simulink model "exportFcnCode"  (R2024b)
settings: Solver=FixedStepAuto  StartTime=0.0  StopTime=10.0  RelTol=1e-3  EnableMultiTasking=on
PostLoadFcn:
  | Variant = 2;
undefined symbols (not defined in the file): CRANK_ANGLE_MAX_IGN, CRANK_ANGLES, cruiseRPM, cyl, duration, dwellAngle, enableCruiseControl, idleRPM, setIgnitionSchedule, timeout, writeCrankAngle, writeCrankRev, writeTotalRevs
libraries: simulink x3
CloseFcn:
  | clear Variant;
settings Model: PauseTimes=74.4  Creator=The MathWorks, Inc.  LastModifiedBy=grouleau
settings SolverCC: AlgebraicLoopSolver=TrustRegion
settings DataIOCC: ReturnWorkspaceOutputs=off
settings OptimizationCC: DefaultParameterBehavior=Inlined  PassReuseOutputArgsAs=Individual arguments  MaxStackSize=64  EfficientTunableParamExpr=on
settings DebuggingCC: ParameterTunabilityLossMsg=error  UnconnectedInputMsg=warning  UnconnectedOutputMsg=warning  UnconnectedLineMsg=warning  PregeneratedLibrarySubsystemCodeDiagnostic=none  ArithmeticOperatorsInVariantConditions=warning
settings HardwareCC: ProdBitPerPointer=32  ProdBitPerSizeT=32  ProdBitPerPtrDiffT=32  ProdLargestAtomicInteger=Long  ProdLargestAtomicFloat=Double  ProdWordSize=32  ProdHWDeviceType=ARM Compatible->ARM Cortex
settings ModelReferenceCC: EnableRefExpFcnMdlSchedulingChecks=on  ModelReferenceNumInstancesAllowed=Single
settings SFSimCC: SimUseLocalCustomCode=off  MATLABDynamicMemAlloc=off  CustomCodeUndefinedFunction=UseInterfaceOnly
settings RTWCC: Description=Embedded Coder  SystemTargetFile=ert.tlc  GenCodeOnly=on  TemplateMakefile=ert_default_tmf  GenerateReport=on  RTWUseLocalCustomCode=off  IncludeHyperlinkInReport=on  LaunchReport=on  GenerateTraceInfo=on  GenerateTraceReport=on  GenerateTraceReportSl=on  GenerateTraceReportSf=on  GenerateTraceReportEml=on  GPUComputeCapability=3.5
settings CodeAppCC: ForceParamTrailComments=on  IgnoreCustomStorageClasses=off  MaxIdLength=63  OperatorAnnotations=on  SimulinkDataObjDesc=on  SFDataObjDesc=on  InsertBlockDesc=on
settings ERTTargetCC: SupportVariableSizeSignals=on  InlinedParameterPlacement=Hierarchical  ERTCustomFileTemplate=example_file_process.tlc  DynamicArrayContainerType=coder::array

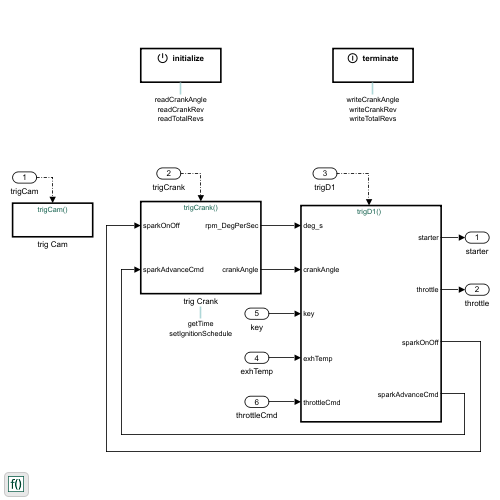
[thumbnail: Simulink's stored preview of the top-level diagram]
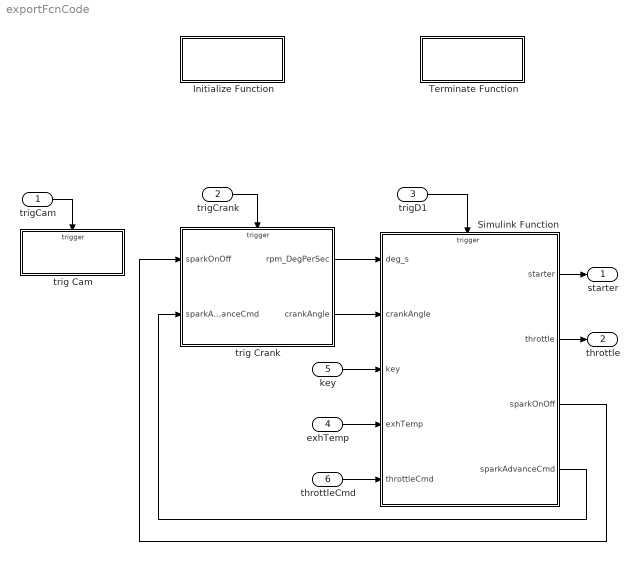
== system exportFcnCode ==
  trigCam : Inport  OutputFunctionCall=on
  trigCrank : Inport  Port=2  OutputFunctionCall=on
  trigD1 : Inport  Port=3  SampleTime=0.008  OutputFunctionCall=on
  exhTemp : Inport  Port=4
  key : Inport  Port=5
  throttleCmd : Inport  Port=6
  Initialize Function : Subsystem  TreatAsAtomicUnit=on
  Simulink Function : Subsystem  TreatAsAtomicUnit=on
  Terminate Function : Subsystem  TreatAsAtomicUnit=on
  trig Cam : Subsystem  TreatAsAtomicUnit=on
  trig Crank : Subsystem  TreatAsAtomicUnit=on
  starter : Outport  VectorParamsAs1DForOutWhenUnconnected=off
  throttle : Outport  Port=2  VectorParamsAs1DForOutWhenUnconnected=off
  wires:
  trig Crank/2(crankAngle) -> Simulink Function/2(crankAngle)
  Simulink Function/2(throttle) -> throttle/1
  Simulink Function/1(starter) -> starter/1
  trigCam/1 -> trig Cam/Trigger
  trig Crank/1(rpm_DegPerSec) -> Simulink Function/1(deg_s)
  key/1 -> Simulink Function/3(key)
  trigCrank/1 -> trig Crank/Trigger
  exhTemp/1 -> Simulink Function/4(exhTemp)
  Simulink Function/3(sparkOnOff) -> trig Crank/1(sparkOnOff)
  Simulink Function/4(sparkAdvanceCmd) -> trig Crank/2(sparkAdvanceCmd)
  trigD1/1 -> Simulink Function/Trigger
  throttleCmd/1 -> Simulink Function/5(throttleCmd)

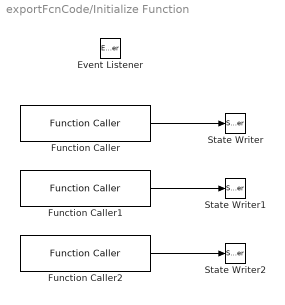
== system exportFcnCode/Initialize Function ==
  Event Listener : EventListener  DisableCoverage=on  EventName=reset
  Function Caller : FunctionCaller  FunctionPrototype=y = readCrankRev()  InputArgumentSpecifications=<Enter example>  OutputArgumentSpecifications=false
  Function Caller1 : FunctionCaller  FunctionPrototype=y = readTotalRevs()  InputArgumentSpecifications=<Enter example>  OutputArgumentSpecifications=0
  Function Caller2 : FunctionCaller  FunctionPrototype=y = readCrankAngle()  InputArgumentSpecifications=<Enter example>  OutputArgumentSpecifications=0
  State Writer : StateWriter  StateOwnerBlock=../../trig Crank/ManageRevolutions/crankRev  StateName=crankRev
  State Writer1 : StateWriter  StateOwnerBlock=../../trig Crank/ManageRevolutions/Total Crank Revolutions  StateName=totalCrankRevs
  State Writer2 : StateWriter  StateOwnerBlock=../../trig Crank/Count Teeth/Local Crank Angle
  wires:
  Function Caller/1 -> State Writer/1
  Function Caller2/1 -> State Writer2/1
  Function Caller1/1 -> State Writer1/1

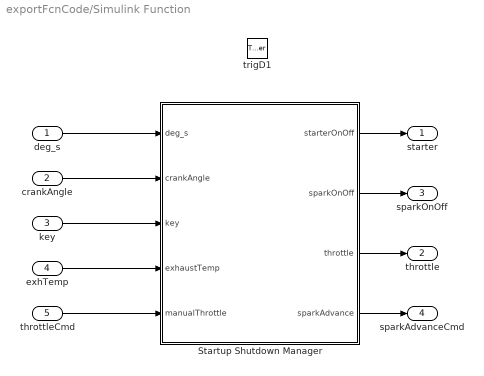
== system exportFcnCode/Simulink Function ==
  deg_s : Inport
  crankAngle : Inport  Port=2
  key : Inport  Port=3
  exhTemp : Inport  Port=4
  throttleCmd : Inport  Port=5
  trigD1 : TriggerPort  TriggerType=function-call  FunctionName=scheduleIgnition  FunctionVisibility=scoped  VariantControl=(inherit)  SampleTimeType=periodic  SampleTime=0.008
  Startup Shutdown Manager : Stateflow chart  TreatAsAtomicUnit=on
  starter : Outport  VectorParamsAs1DForOutWhenUnconnected=off
  throttle : Outport  Port=2  VectorParamsAs1DForOutWhenUnconnected=off
  sparkOnOff : Outport  Port=3  VectorParamsAs1DForOutWhenUnconnected=off
  sparkAdvanceCmd : Outport  Port=4  VectorParamsAs1DForOutWhenUnconnected=off
  wires:
  crankAngle/1 -> Startup Shutdown Manager/2(crankAngle)
  deg_s/1 -> Startup Shutdown Manager/1(deg_s)
  key/1 -> Startup Shutdown Manager/3(key)
  Startup Shutdown Manager/1(starterOnOff) -> starter/1
  Startup Shutdown Manager/2(sparkOnOff) -> sparkOnOff/1
  Startup Shutdown Manager/3(throttle) -> throttle/1
  exhTemp/1 -> Startup Shutdown Manager/4(exhaustTemp)
  Startup Shutdown Manager/4(sparkAdvance) -> sparkAdvanceCmd/1
  throttleCmd/1 -> Startup Shutdown Manager/5(manualThrottle)

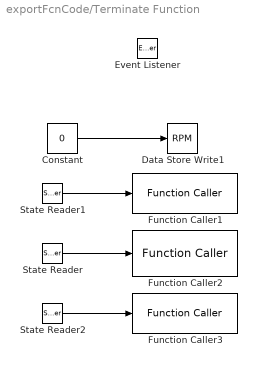
== system exportFcnCode/Terminate Function ==
  Constant : Constant  Value=0
  Data Store Write1 : DataStoreWrite  DataStoreName=RPM  IndexOptions=Index vector (dialog)  Indices=1  OutputSizes=1
  Event Listener : EventListener  DisableCoverage=on  EventType=Terminate  EventName=reset
  Function Caller1 : FunctionCaller  FunctionPrototype=writeCrankRev(u)  InputArgumentSpecifications=false  OutputArgumentSpecifications=<Enter example>
  Function Caller2 : FunctionCaller  FunctionPrototype=writeTotalRevs(u)  InputArgumentSpecifications=0  OutputArgumentSpecifications=<Enter example>
  Function Caller3 : FunctionCaller  FunctionPrototype=writeCrankAngle(u)  InputArgumentSpecifications=0  OutputArgumentSpecifications=<Enter example>
  State Reader : StateReader  StateOwnerBlock=../../trig Crank/ManageRevolutions/Total Crank Revolutions  StateName=totalCrankRevs
  State Reader1 : StateReader  StateOwnerBlock=../../trig Crank/ManageRevolutions/crankRev  StateName=crankRev
  State Reader2 : StateReader  StateOwnerBlock=../../trig Crank/Count Teeth/Local Crank Angle
  wires:
  State Reader/1 -> Function Caller2/1
  Constant/1 -> Data Store Write1/1
  State Reader2/1 -> Function Caller3/1
  State Reader1/1 -> Function Caller1/1

== system exportFcnCode/trig Cam ==
  trigCam : TriggerPort  TriggerType=function-call  FunctionName=trigCam  FunctionVisibility=scoped  VariantControl=(inherit)
  Constant : Constant  Value=false
  State Writer : StateWriter  StateOwnerBlock=../../trig Crank/ManageRevolutions/crankRev  StateName=crankRev
  wires:
  Constant/1 -> State Writer/1

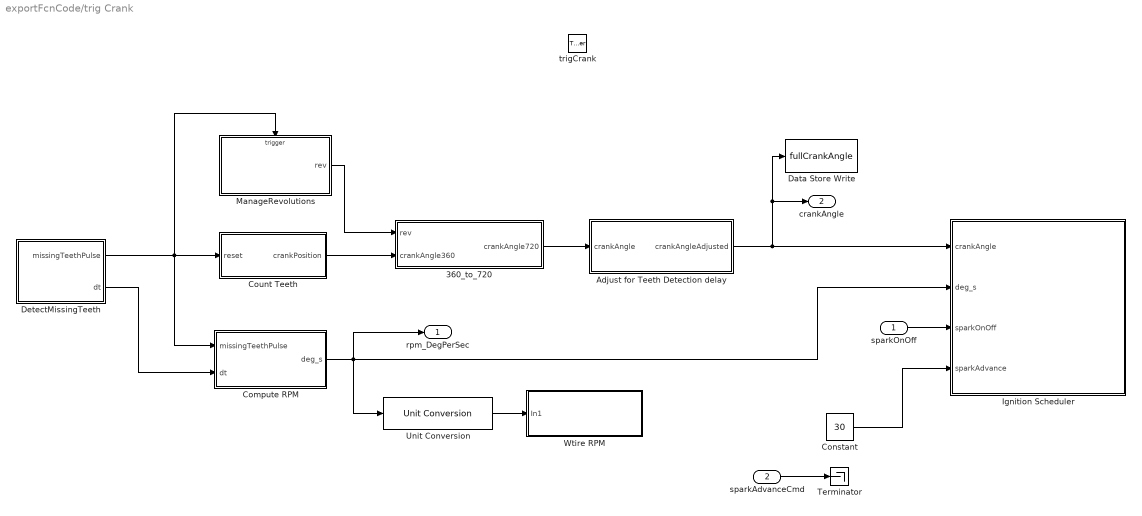
== system exportFcnCode/trig Crank ==
  sparkOnOff : Inport
  sparkAdvanceCmd : Inport  Port=2
  trigCrank : TriggerPort  TriggerType=function-call  FunctionName=trigCrank  FunctionVisibility=scoped  VariantControl=(inherit)
  360_to_720 : Subsystem
  Adjust for Teeth Detection delay : Subsystem
  Compute RPM : Subsystem
  Constant : Constant  Value=30
  Count Teeth : Subsystem
  Data Store Write : DataStoreWrite  DataStoreName=fullCrankAngle  IndexOptions=Index vector (dialog)  Indices=1  OutputSizes=1
  DetectMissingTeeth : Subsystem
  Ignition Scheduler : Stateflow chart  TreatAsAtomicUnit=on
  ManageRevolutions : Subsystem
  Terminator : Terminator
  Unit Conversion : UnitConversion
  Wtire RPM : Subsystem
  rpm_DegPerSec : Outport  VectorParamsAs1DForOutWhenUnconnected=off
  crankAngle : Outport  Port=2  VectorParamsAs1DForOutWhenUnconnected=off
  wires:
  360_to_720/1(crankAngle720) -> Adjust for Teeth Detection delay/1(crankAngle)
  Count Teeth/1(crankPosition) -> 360_to_720/2(crankAngle360)
  DetectMissingTeeth/1(missingTeethPulse) -> ManageRevolutions/Trigger, Compute RPM/1(missingTeethPulse), Count Teeth/1(reset)
  DetectMissingTeeth/2(dt) -> Compute RPM/2(dt)
  Compute RPM/1(deg_s) -> Ignition Scheduler/2(deg_s), Unit Conversion/1, rpm_DegPerSec/1
  Adjust for Teeth Detection delay/1(crankAngleAdjusted) -> Data Store Write/1, crankAngle/1, Ignition Scheduler/1(crankAngle)
  Unit Conversion/1 -> Wtire RPM/1(In1)
  sparkOnOff/1 -> Ignition Scheduler/3(sparkOnOff)
  ManageRevolutions/1(rev) -> 360_to_720/1(rev)
  Constant/1 -> Ignition Scheduler/4(sparkAdvance)
  sparkAdvanceCmd/1 -> Terminator/1

== system exportFcnCode/Simulink Function/Startup Shutdown Manager/ManageStartupShutdown.exhausttempCtrl ==
  exhTemp : Inport  OutDataTypeStr=double  PortDimensions=1
  f : TriggerPort  TriggerType=function-call  VariantControl=(inherit)
      settings: CopyFcn=Stateflow.SLINSF.SimulinkMan.removeBlockPreDeleteFcn  PreDeleteFcn=Stateflow.SLINSF.SimulinkMan.unsafePredeleteFcn
  1-D Lookup Table : Lookup_n-D  NumberOfTableDimensions=1  BreakpointsForDimension1=[25 50 75 100 150]  Table=[10 10 10 20 20]  ExtrapMethod=Clip  InternalRulePriority=Speed  RndMeth=Simplest
  sparkAdvance : Outport  VectorParamsAs1DForOutWhenUnconnected=off
  wires:
  exhTemp/1 -> 1-D Lookup Table/1
  1-D Lookup Table/1 -> sparkAdvance/1

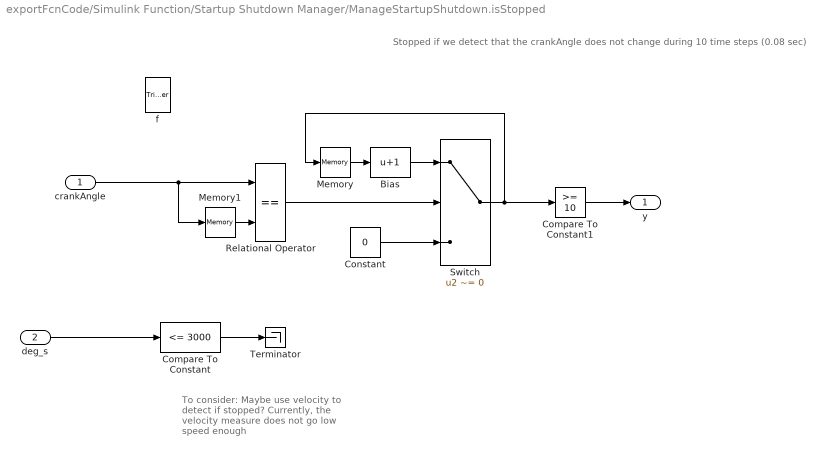
== system exportFcnCode/Simulink Function/Startup Shutdown Manager/ManageStartupShutdown.isStopped ==
  note: Stopped if we detect that the crankAngle does not change during 10 time steps (0.08 sec)
  note: To consider:
      | Maybe use velocity to detect if stopped?
      | Currently, the velocity measure does not go low speed enough
  crankAngle : Inport  OutDataTypeStr=double  PortDimensions=1
  deg_s : Inport  Port=2  OutDataTypeStr=double  PortDimensions=1
  f : TriggerPort  TriggerType=function-call  VariantControl=(inherit)
      settings: CopyFcn=Stateflow.SLINSF.SimulinkMan.removeBlockPreDeleteFcn  PreDeleteFcn=Stateflow.SLINSF.SimulinkMan.unsafePredeleteFcn
  Bias : Bias  Bias=1  SaturateOnIntegerOverflow=off
  Compare To Constant : simulink/Logic and Bit Operations/Compare To Constant  relop=<=  const=3000  OutDataTypeStr=boolean
  Compare To Constant1 : simulink/Logic and Bit Operations/Compare To Constant  relop=>=  const=10  OutDataTypeStr=boolean
  Constant : Constant  Value=0
  Memory : Memory  InheritSampleTime=on
  Memory1 : Memory  InheritSampleTime=on
  Relational Operator : RelationalOperator  Operator===  OutDataTypeStr=boolean  RndMeth=Simplest  InputSameDT=off
  Switch : Switch  Criteria=u2 ~= 0  SaturateOnIntegerOverflow=off  InputSameDT=off
  Terminator : Terminator
  y : Outport  OutDataTypeStr=boolean  PortDimensions=1  VectorParamsAs1DForOutWhenUnconnected=off
  wires:
  deg_s/1 -> Compare To Constant/1
  Switch/1 -> Compare To Constant1/1, Memory/1
  Memory/1 -> Bias/1
  Relational Operator/1 -> Switch/2
  crankAngle/1 -> Memory1/1, Relational Operator/1
  Bias/1 -> Switch/1
  Constant/1 -> Switch/3
  Memory1/1 -> Relational Operator/2
  Compare To Constant1/1 -> y/1
  Compare To Constant/1 -> Terminator/1

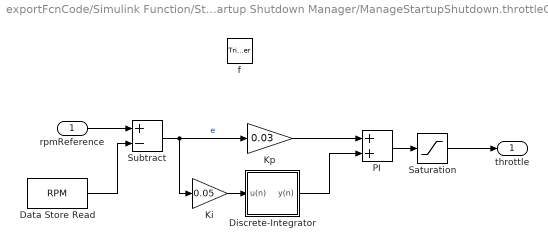
== system exportFcnCode/Simulink Function/Startup Shutdown Manager/ManageStartupShutdown.throttleControl ==
  rpmReference : Inport  OutDataTypeStr=double  PortDimensions=1
  f : TriggerPort  TriggerType=function-call  VariantControl=(inherit)
      settings: CopyFcn=Stateflow.SLINSF.SimulinkMan.removeBlockPreDeleteFcn  PreDeleteFcn=Stateflow.SLINSF.SimulinkMan.unsafePredeleteFcn
  Data Store Read : DataStoreRead  DataStoreName=RPM  IndexOptions=Index vector (dialog)  Indices=1  OutputSizes=1
  Discrete-Integrator : Subsystem
  Ki : Gain  Gain=0.05
  Kp : Gain  Gain=0.03
  PI : Sum
  Saturation : Saturate  UpperLimit=90  LowerLimit=0
  Subtract : Sum  Inputs=+-
  throttle : Outport  VectorParamsAs1DForOutWhenUnconnected=off
  wires:
  rpmReference/1 -> Subtract/1
  Data Store Read/1 -> Subtract/2
  Subtract/1 -> Kp/1, Ki/1  "e"
  Discrete-Integrator/1(y(n)) -> PI/2
  PI/1 -> Saturation/1
  Ki/1 -> Discrete-Integrator/1(u(n))
  Kp/1 -> PI/1
  Saturation/1 -> throttle/1

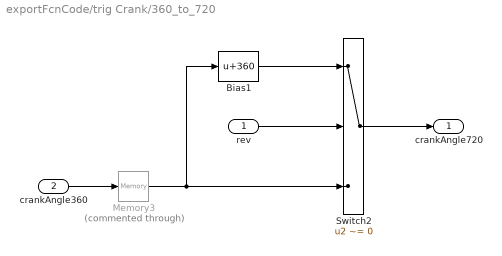
== system exportFcnCode/trig Crank/360_to_720 ==
  rev : Inport
  crankAngle360 : Inport  Port=2
  Bias1 : Bias  Bias=360  SaturateOnIntegerOverflow=off
  Memory3 : Memory  Commented=through  InheritSampleTime=on
  Switch2 : Switch  Criteria=u2 ~= 0  Threshold=34  SaturateOnIntegerOverflow=off  InputSameDT=off
  crankAngle720 : Outport  VectorParamsAs1DForOutWhenUnconnected=off
  wires:
  rev/1 -> Switch2/2
  Switch2/1 -> crankAngle720/1
  Bias1/1 -> Switch2/1
  Memory3/1 -> Bias1/1, Switch2/3
  crankAngle360/1 -> Memory3/1

== system exportFcnCode/trig Crank/Adjust for Teeth Detection delay ==
  crankAngle : Inport
  Bias2 : Bias  Commented=through  Bias=10  SaturateOnIntegerOverflow=off
  Bias3 : Bias  Bias=-710  SaturateOnIntegerOverflow=off
  Compare To Constant1 : simulink/Logic and Bit Operations/Compare To Constant  relop=>  const=700  OutDataTypeStr=boolean
  Switch3 : Switch  Criteria=u2 ~= 0  Threshold=34  SaturateOnIntegerOverflow=off  InputSameDT=off
  crankAngleAdjusted : Outport  VectorParamsAs1DForOutWhenUnconnected=off
  wires:
  Switch3/1 -> crankAngleAdjusted/1  "crankAngleAdjusted"
  Compare To Constant1/1 -> Switch3/2
  Bias2/1 -> Switch3/3, Compare To Constant1/1, Bias3/1
  crankAngle/1 -> Bias2/1
  Bias3/1 -> Switch3/1

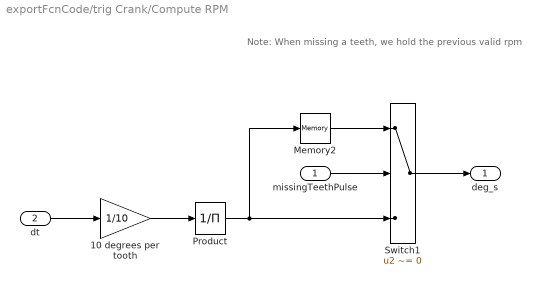
== system exportFcnCode/trig Crank/Compute RPM ==
  note: Note: When missing a teeth, we hold the previous valid rpm
  missingTeethPulse : Inport
  dt : Inport  Port=2  Unit=sec
  10 degrees per tooth : Gain  Gain=1/10
  Memory2 : Memory  InheritSampleTime=on
  Product : Product  Inputs=/
  Switch1 : Switch  Criteria=u2 ~= 0  Threshold=34  SaturateOnIntegerOverflow=off  InputSameDT=off
  deg_s : Outport  Unit=deg/sec  VectorParamsAs1DForOutWhenUnconnected=off
  wires:
  10 degrees per tooth/1 -> Product/1
  Product/1 -> Memory2/1, Switch1/3
  Memory2/1 -> Switch1/1
  Switch1/1 -> deg_s/1
  dt/1 -> 10 degrees per tooth/1
  missingTeethPulse/1 -> Switch1/2

== system exportFcnCode/trig Crank/Count Teeth ==
  note: Crank Position 0-360
  reset : Inport
  Bias : Bias  Bias=10  SaturateOnIntegerOverflow=off
  Constant1 : Constant  Value=0
  Local Crank Angle : UnitDelay  SampleTime=-1  HasFrameUpgradeWarning=on
  Switch : Switch  Criteria=u2 ~= 0  Threshold=34  SaturateOnIntegerOverflow=off  InputSameDT=off
  crankPosition : Outport  Unit=deg  VectorParamsAs1DForOutWhenUnconnected=off
  wires:
  Constant1/1 -> Switch/1
  reset/1 -> Switch/2
  Switch/1 -> Local Crank Angle/1, crankPosition/1
  Local Crank Angle/1 -> Bias/1
  Bias/1 -> Switch/3

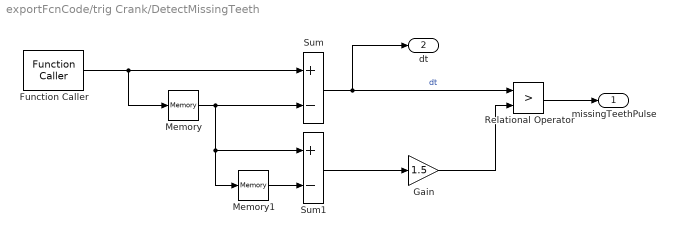
== system exportFcnCode/trig Crank/DetectMissingTeeth ==
  Function Caller : FunctionCaller  FunctionPrototype=y = getTime()  InputArgumentSpecifications=<Enter example>  OutputArgumentSpecifications=1
  Gain : Gain  Gain=1.5
  Memory : Memory  InheritSampleTime=on
  Memory1 : Memory  InheritSampleTime=on
  Relational Operator : RelationalOperator  Operator=>  OutDataTypeStr=boolean  RndMeth=Simplest  InputSameDT=off
  Sum : Sum  Inputs=+-
  Sum1 : Sum  Inputs=+-
  missingTeethPulse : Outport  VectorParamsAs1DForOutWhenUnconnected=off
  dt : Outport  Port=2  Unit=sec  VectorParamsAs1DForOutWhenUnconnected=off
  wires:
  Sum/1 -> dt/1, Relational Operator/1  "dt"
  Function Caller/1 -> Memory/1, Sum/1
  Memory/1 -> Sum1/1, Memory1/1, Sum/2
  Memory1/1 -> Sum1/2
  Relational Operator/1 -> missingTeethPulse/1
  Gain/1 -> Relational Operator/2
  Sum1/1 -> Gain/1

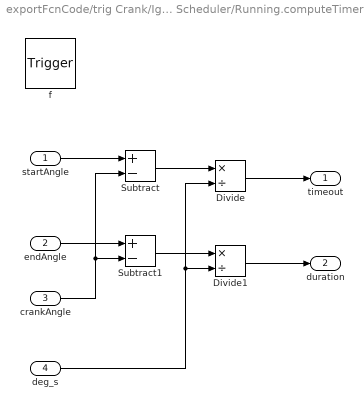
== system exportFcnCode/trig Crank/Ignition Scheduler/Running.computeTimerProps ==
  startAngle : Inport  OutDataTypeStr=double  PortDimensions=1
  endAngle : Inport  Port=2  OutDataTypeStr=double  PortDimensions=1
  crankAngle : Inport  Port=3  OutDataTypeStr=double  PortDimensions=1
  deg_s : Inport  Port=4  OutDataTypeStr=double  PortDimensions=1
  f : TriggerPort  TriggerType=function-call  VariantControl=(inherit)
      settings: CopyFcn=Stateflow.SLINSF.SimulinkMan.removeBlockPreDeleteFcn  PreDeleteFcn=Stateflow.SLINSF.SimulinkMan.unsafePredeleteFcn
  Divide : Product  Inputs=*/
  Divide1 : Product  Inputs=*/
  Subtract : Sum  Inputs=+-
  Subtract1 : Sum  Inputs=+-
  timeout : Outport  VectorParamsAs1DForOutWhenUnconnected=off
  duration : Outport  Port=2  VectorParamsAs1DForOutWhenUnconnected=off
  wires:
  startAngle/1 -> Subtract/1
  crankAngle/1 -> Subtract1/2, Subtract/2
  endAngle/1 -> Subtract1/1
  Subtract/1 -> Divide/1
  deg_s/1 -> Divide1/2, Divide/2
  Subtract1/1 -> Divide1/1
  Divide1/1 -> duration/1
  Divide/1 -> timeout/1

== system exportFcnCode/trig Crank/Ignition Scheduler/Running.setIgnitionScheduleWrapper ==
  cyl : Inport  OutDataTypeStr=double  PortDimensions=1
  timeout : Inport  Port=2  OutDataTypeStr=double  PortDimensions=1
  duration : Inport  Port=3  OutDataTypeStr=double  PortDimensions=1
  f : TriggerPort  TriggerType=function-call  VariantControl=(inherit)
      settings: CopyFcn=Stateflow.SLINSF.SimulinkMan.removeBlockPreDeleteFcn  PreDeleteFcn=Stateflow.SLINSF.SimulinkMan.unsafePredeleteFcn
  Function Caller : FunctionCaller  FunctionPrototype=setIgnitionSchedule(cyl,timeout,duration)  InputArgumentSpecifications=1,1,1  OutputArgumentSpecifications=<Enter example>
  wires:
  cyl/1 -> Function Caller/1
  timeout/1 -> Function Caller/2
  duration/1 -> Function Caller/3

== system exportFcnCode/trig Crank/ManageRevolutions ==
  Trigger : TriggerPort  VariantControl=Variant  PortDimensions=1
  Bias : Bias  Bias=1  SaturateOnIntegerOverflow=off
  NOT : Logic  Operator=NOT  IconShape=distinctive  AllPortsSameDT=off  OutDataTypeStr=boolean
  Total Crank Revolutions : UnitDelay  SampleTime=-1  StateName=totalCrankRevs  HasFrameUpgradeWarning=on
  crankRev : UnitDelay  InitialCondition=false  SampleTime=-1  StateName=crankRev  HasFrameUpgradeWarning=on
  rev : Outport  VectorParamsAs1DForOutWhenUnconnected=off
  wires:
  crankRev/1 -> NOT/1
  NOT/1 -> rev/1, crankRev/1
  Bias/1 -> Total Crank Revolutions/1
  Total Crank Revolutions/1 -> Bias/1

== system exportFcnCode/trig Crank/Wtire RPM ==
  In1 : Inport  Unit=rpm
  Data Store Write1 : DataStoreWrite  DataStoreName=RPM  IndexOptions=Index vector (dialog)  Indices=1  OutputSizes=1
  wires:
  In1/1 -> Data Store Write1/1

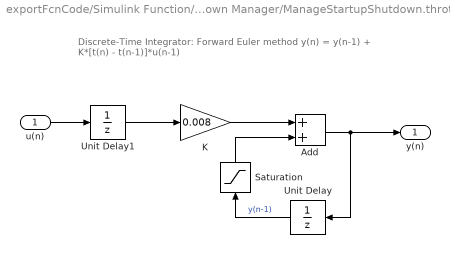
== system exportFcnCode/Simulink Function/Startup Shutdown Manager/ManageStartupShutdown.throttleControl/Discrete-Integrator ==
  note: Discrete-Time Integrator: Forward Euler method
      | y(n) = y(n-1) + K*[t(n) - t(n-1)]*u(n-1)
  u(n) : Inport
  Add : Sum
  K : Gain  Gain=0.008
  Saturation : Saturate  UpperLimit=90  LowerLimit=0
  Unit Delay : UnitDelay  SampleTime=-1  HasFrameUpgradeWarning=on
  Unit Delay1 : UnitDelay  SampleTime=-1  HasFrameUpgradeWarning=on
  y(n) : Outport  VectorParamsAs1DForOutWhenUnconnected=off
  wires:
  K/1 -> Add/1
  Unit Delay1/1 -> K/1
  Add/1 -> y(n)/1, Unit Delay/1
  u(n)/1 -> Unit Delay1/1
  Unit Delay/1 -> Saturation/1  "y(n-1)"
  Saturation/1 -> Add/2

== stateflow chart exportFcnCode/Simulink Function/Startup Shutdown Manager ==
  settings: sampleTime=0.008
  state ManageStartupShutdown [parallel]
    settings: executionOrder=1
    state Off
      entry: starterOnOff = false;
      sparkOnOff = false;
      throttle = 0;
    state Running
      state StarterOn
        entry: starterOnOff = true;
      state SparkOn
        entry: sparkOnOff = true;
        throttle = 90;
      state StarterAndEngine
      state StarterOff
        entry:
        starterOnOff = false;
        entry, during:
        if(enableCruiseControl)
        throttle = throttleControl(cruiseRPM);
        else
        throttle = manualThrottle+throttleControl(idleRPM);
        end
        sparkAdvance = exhausttempCtrl(exhaustTemp);
      (default) -> StarterOn
      StarterOn -> SparkOn : after(0.5,sec)
      SparkOn -> StarterAndEngine
      StarterAndEngine -> StarterOff : [deg_s>10000] % over 1600 RPM
    state WaitingForZeroSped
    state throttle = throttleControl(rpmReference) [function]
    state y = isStopped(crankAngle,deg_s) [function]
    state sparkAdvance = exhausttempCtrl(exhTemp) [function]
    (default) -> Off
    (junction 242) -> Off
    (junction 241) -> (junction 242) : [isStopped(crankAngle,deg_s)]
        | {isECUPowered = false;}
    Off -> Running : [key == true]
    Running -> WaitingForZeroSped : [key == false]
        | {throttle = 0;sparkOnOff=false}
    WaitingForZeroSped -> (junction 241)
  data: throttle function_output; rpmReference function_input double size=1; crankAngle function_input double size=1; deg_s function_input double size=1; y function_output boolean size=1; exhTemp function_input double size=1; sparkAdvance function_output; deg_s input; dwellAngle parameter; crankAngle input; CRANK_ANGLES parameter; key input boolean size=1; starterOnOff output boolean size=1; sparkOnOff output boolean size=1; throttle output double size=1; isECUPowered data_store_memory; enableCruiseControl parameter; cruiseRPM parameter; exhaustTemp input; idleRPM parameter; sparkAdvance output; manualThrottle input

== stateflow chart exportFcnCode/trig Crank/Ignition Scheduler ==
  state Wait
  state Running
    state [timeout, duration] = computeTimerProps(startAngle, endAngle, crankAngle, deg_s) [function]
    state setIgnitionScheduleWrapper(cyl,timeout,duration) [function]
    state WaitNextQuadrant
    note: CRANK_ANGLES = [720 180 360 540];
    state startAt1
      en:  endAngle = CRANK_ANGLES(1) - sparkAdvance;
      startAngle = endAngle-dwellAngle;
    state IgnitionCyl1
      entry: [timeout, duration] = computeTimerProps(startAngle, endAngle, crankAngle, deg_s);
      setIgnitionScheduleWrapper(1,timeout,duration);
      endAngle = CRANK_ANGLES(2) - sparkAdvance;
      startAngle = endAngle-dwellAngle;
    state IgnitionCyl2
      entry: [timeout, duration] = computeTimerProps(startAngle, endAngle, crankAngle, deg_s);
      setIgnitionScheduleWrapper(2,timeout,duration);
      endAngle = CRANK_ANGLES(3) - sparkAdvance;
      startAngle = endAngle-dwellAngle;
    state startAt2
      en:  endAngle = CRANK_ANGLES(2) - sparkAdvance;
      startAngle = endAngle-dwellAngle;
    state IgnitionCyl3
      entry: [timeout, duration] = computeTimerProps(startAngle, endAngle, crankAngle, deg_s);
      setIgnitionScheduleWrapper(3,timeout,duration);
      endAngle = CRANK_ANGLES(4) - sparkAdvance;
      startAngle = endAngle-dwellAngle;
    state startAt3
      en:  endAngle = CRANK_ANGLES(3) - sparkAdvance;
      startAngle = endAngle-dwellAngle;
    state IgnitionCyl4
      entry: [timeout, duration] = computeTimerProps(startAngle, endAngle, crankAngle, deg_s);
      setIgnitionScheduleWrapper(4,timeout,duration);
      endAngle = CRANK_ANGLES(1) - sparkAdvance;
      startAngle = endAngle-dwellAngle;
    state startAt4
      en:  endAngle = CRANK_ANGLES(4) - sparkAdvance;
      startAngle = endAngle-dwellAngle;
    (default) -> WaitNextQuadrant
    WaitNextQuadrant -> (junction 141)
    (junction 141) -> (junction 162) [order 1]
    (junction 141) -> (junction 137) [order 2]
    (junction 162) -> startAt1 : [crankAngle >= CRANK_ANGLES(3) && crankAngle < CRANK_ANGLES(4) ] % We are in 3rd quadrant
    startAt1 -> IgnitionCyl1 : [crankAngle > CRANK_ANGLES(4)]
        | % We enter 4th quadrant
    (junction 130) -> IgnitionCyl1
    (junction 128) -> (junction 130)
    IgnitionCyl1 -> IgnitionCyl2 : [crankAngle < CRANK_ANGLES(2)  ]% We passed zero
    (junction 137) -> (junction 115) [order 1]
    (junction 137) -> (junction 129) [order 2]
    (junction 115) -> startAt2 : [crankAngle >= CRANK_ANGLES(4) && crankAngle < CRANK_ANGLES(1) ]	% We are in 4th quadrant
    startAt2 -> IgnitionCyl2 : [crankAngle < CRANK_ANGLES(2)  ]
        | % We enter 1st quadrant
    IgnitionCyl2 -> IgnitionCyl3 : [crankAngle > CRANK_ANGLES(2)  ]	%  We passed 180
    (junction 129) -> (junction 168) [order 1]
    (junction 168) -> startAt3 : [crankAngle < CRANK_ANGLES(2)] % We are in 1st quadrant
    (junction 129) -> (junction 109) [order 2]
    startAt3 -> IgnitionCyl3 : [crankAngle > CRANK_ANGLES(2) ]
        | % We enter 2nd quadrant
    IgnitionCyl3 -> IgnitionCyl4 : [crankAngle > CRANK_ANGLES(3)  ] % We passed 360
    (junction 109) -> (junction 131)
    (junction 131) -> startAt4 : [crankAngle < CRANK_ANGLES(3)  ] % We are in 2nd quadrant
    startAt4 -> IgnitionCyl4 : [crankAngle > CRANK_ANGLES(3)  ]
        | % We enter 3rd quadrant
    IgnitionCyl4 -> (junction 107) : [crankAngle > CRANK_ANGLES(4)  ] % We passed 540
    (junction 107) -> (junction 128)
  (default) -> Wait
  Wait -> Running : [sparkOnOff==1]
  Running -> Wait : [sparkOnOff==0]
  data: startAngle function_input double size=1; endAngle function_input double size=1; crankAngle function_input double size=1; deg_s function_input double size=1; timeout function_output; duration function_output; cyl function_input double size=1; timeout function_input double size=1; duration function_input double size=1; startAngle local; endAngle local; dwellAngle parameter; CRANK_ANGLE_MAX_IGN parameter; CRANK_ANGLES parameter; duration local; timeout local; crankAngle input double size=1; deg_s input; sparkOnOff input; sparkAdvance input
